simulink model "G431_ADC_Converter"  (R2018b)
settings: Solver=FixedStepDiscrete  StartTime=0.0  StopTime=10.0  FixedStep=0.010  RelTol=1e-3  EnableMultiTasking=on
settings Model: Creator=reynaudp  LastModifiedBy=fenard1
settings DataIOCC: LimitDataPoints=on  SaveFormat=Array  SaveOutput=off  SaveTime=off
settings OptimizationCC: DefaultParameterBehavior=Inlined  DefaultUnderspecifiedDataType=single  LifeSpan=1
settings DebuggingCC: UnderspecifiedInitializationDetection=Classic  MergeDetectMultiDrivingBlocksExec=none  SolverPrmCheckMsg=warning  UniqueDataStoreMsg=error  AllowSymbolicDim=off  StrictBusMsg=ErrorOnBusTreatedAsVector  SFUnexpectedBacktrackingDiag=warning  SFNoUnconditionalDefaultTransitionDiag=warning  SFUndirectedBroadcastEventsDiag=error  SFExecutionAtInitializationDiag=none
settings HardwareCC: ProdBitPerPointer=32  ProdBitPerSizeT=32  ProdBitPerPtrDiffT=32  ProdLargestAtomicInteger=Integer  ProdWordSize=32  ProdHWDeviceType=STMicroelectronics->STM32 32-bit Cortex-M  TargetBitPerPointer=64  TargetBitPerSizeT=64  TargetBitPerPtrDiffT=64  TargetLongLongMode=on  TargetIntDivRoundTo=Zero  TargetEndianess=LittleEndian  TargetWordSize=64  TargetHWDeviceType=MATLAB Host  ProdEqTarget=off
settings ModelReferenceCC: PropagateSignalLabelsOutOfModel=off
settings SFSimCC: SimUseLocalCustomCode=off  CompileTimeRecursionLimit=0  EnableRuntimeRecursion=off  MATLABDynamicMemAlloc=off
settings RTWCC: SystemTargetFile=stm32.tlc  TemplateMakefile=stm32.tmf  Description=stm32 (Embedded Target)  GenerateReport=on  RTWUseLocalCustomCode=off  IncludeHyperlinkInReport=on
settings CodeAppCC: IgnoreCustomStorageClasses=off  CustomSymbolStrType=$N$R$M  SimulinkBlockComments=off
settings STFCustomTargetCC: ParMdlRefBuildCompliant=on  IncludeMdlTerminateFcn=off  CombineOutputUpdateFcns=on  ERTCustomFileBanners=on  SupportComplex=off  SupportContinuousTime=off  SupportNonInlinedSFcns=off  RemoveResetFunc=on  CastingMode=Standards  MATLABClassNameForMDSCustomization=Simulink.SoftwareTarget.ERTCustomization  SystemTargetFile=stm32.tlc
settings ERTTargetCC: MultiwordLength=2048  CompOptLevelCompliant=off  ConcurrentExecutionCompliant=off  IncludeMdlTerminateFcn=off  SupportComplex=off  CastingMode=Standards  ModelStepFunctionPrototypeControlCompliant=off  CPPClassGenCompliant=off  UseToolchainInfoCompliant=off  ERTSrcFileBannerTemplate=sourceFileTemplate.cgt  ERTHdrFileBannerTemplate=sourceFileTemplate.cgt  ERTDataSrcFileTemplate=sourceFileTemplate.cgt  ERTDataHdrFileTemplate=sourceFileTemplate.cgt  ERTCustomFileTemplate=customRoutineProcess.tlc  ConvertIfToSwitch=off  SuppressUnreachableDefaultCases=off
settings ConfigComp: CovMetricSettings=dw  CovHtmlReporting=on  CovSaveCumulativeToWorkspaceVar=on  CovSaveSingleToWorkspaceVar=on  CovExternalEMLEnable=off  CovSFcnEnable=off

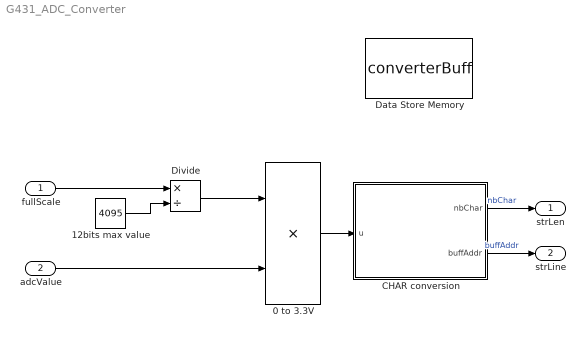
== system G431_ADC_Converter ==
  fullScale : Inport  OutDataTypeStr=double  PortDimensions=1
  adcValue : Inport  Port=2  OutDataTypeStr=double  PortDimensions=1  SampleTime=[0.20000000000000001,0]
  0 to 3.3V : Product  RndMeth=Zero
  12bits max value : Constant  Value=4095
  CHAR conversion : MATLAB Function  TreatAsAtomicUnit=on  SystemSampleTime=0.200
      settings: AttributesFormatString=SystemSampleTime=%<SystemSampleTime>
  Data Store Memory : DataStoreMemory  DataStoreName=converterBuff  ReadBeforeWriteMsg=warning  WriteAfterWriteMsg=warning  WriteAfterReadMsg=warning  InitialValue=[0,0,0,0,0,0,0,0,0,0,0,0,0,0,0,0,0,0,0,0,0,0,0,0,0,0,0]  ShowAdditionalParam=off  OutDataTypeStr=uint8
  Divide : Product  Inputs=*/
  strLen : Outport  OutDataTypeStr=uint16  PortDimensions=1  SampleTime=[0.20000000000000001,0]
  strLine : Outport  Port=2  OutDataTypeStr=uint32  PortDimensions=1  SampleTime=[0.20000000000000001,0]
  wires:
  CHAR conversion/2(buffAddr) -> strLine/1  "buffAddr"
  0 to 3.3V/1 -> CHAR conversion/1(u)
  adcValue/1 -> 0 to 3.3V/2
  fullScale/1 -> Divide/1
  CHAR conversion/1(nbChar) -> strLen/1  "nbChar"
  Divide/1 -> 0 to 3.3V/1
  12bits max value/1 -> Divide/2

== matlab function G431_ADC_Converter/CHAR conversion ==
  data: u input; nbChar output uint16 size=1; buffAddr output uint32 size=1; converterBuff data_store_memory
function [nbChar, buffAddr] = convert(u) %#codegen
global converterBuff;

if coder.target('Sfun')
    % Executing in MATLAB, Buff is null
    buffAddr = uint32(0);
    nbChar = uint16(0);
else
    coder.cinclude('stdio.h');
    coder.cinclude('main.h');
    coder.cinclude('getBuffPtr.h');
    % Executing in the generated code.
    %%%converterBuff = char(zeros(1,20));
    %%%stringSize = uint16(size(converterBuff,2));
    stringSize = uint16(20);
    stringFormat = char(['%08x-%5.2f V',13,10,0]);
    tick = uint32(0);
    tick = coder.ceval('HAL_GetTick');
    nbChar = coder.ceval('-global','snprintf',coder.wref(converterBuff),stringSize,coder.rref(stringFormat),tick,u);
    buffAddr = coder.ceval('-global','getBuffPtr',coder.rref(converterBuff));
end
end
